simulink model "BlokSchema3 - Older"  (R2022a)
settings: Solver=VariableStepAuto  StartTime=0.0  StopTime=5000  RelTol=1e-5
values from neighbouring files (symbols this model uses):
  citatel = (K/(T1*T2))    (= 0.00186096256684)    [Zadanie3.m]    (also in Zadanie3_v2.m)
  Delay = 300    [Zadanie3.m]    (also in Zadanie3_v2.m)
  menovatel = [1,(T1+T2)/(T1*T2), 1/(T1*T2)]    [Zadanie3.m]    (also in Zadanie3_v2.m)
  p01 = citatel1(2)*q00    [Zadanie3.m]    (also in Zadanie3_v2.m)
  p02 = citatel1(3)*q00    [Zadanie3.m]    (also in Zadanie3_v2.m)
  p03 = citatel1(4)*q00    [Zadanie3_v2.m]
  p11 = q10*citatel1(2)    [Zadanie3.m]    (also in Zadanie3_v2.m)
  p12 = q10*(citatel1(3)-citatel1(2))+(citatel1(2)/bSum)    [Zadanie3.m]    (also in Zadanie3_v2.m)
  p13 = q10*(citatel1(4)-citatel1(3))+(citatel1(3)/bSum)    [Zadanie3.m]    (also in Zadanie3_v2.m)
  q00 = 1/sum(citatel1(2:end))    [Zadanie3.m]    (also in Zadanie3_v2.m)
  q01 = menovatel1(2)*q00    [Zadanie3.m]    (also in Zadanie3_v2.m)
  q02 = menovatel1(3)*q00    [Zadanie3.m]    (also in Zadanie3_v2.m)
  q03 = menovatel1(4)*q00    [Zadanie3_v2.m]
  q10 = 0.089115984    [Zadanie3.m]    (also in Zadanie3_v2.m)
  q11 = q10*(menovatel1(2)-1)+1/bSum    [Zadanie3.m]    (also in Zadanie3_v2.m)
  q12 = q10*(menovatel1(3)-menovatel1(2))+(menovatel1(2)/bSum)    [Zadanie3.m]    (also in Zadanie3_v2.m)
  q13 = q10*(menovatel1(4)-menovatel1(3))+(menovatel1(3)/bSum)    [Zadanie3.m]    (also in Zadanie3_v2.m)
  T = 300    [Zadanie3.m]    (also in Zadanie3_v2.m)
settings Model: PacingRate=100  Creator=domin  LastModifiedBy=domin
settings ModelReferenceCC: EnableRefExpFcnMdlSchedulingChecks=off
settings RTWCC: Description=Generic Real-Time Target

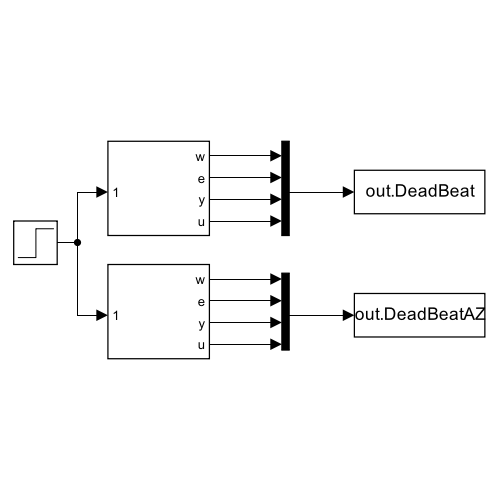
[thumbnail: Simulink's stored preview of the top-level diagram]
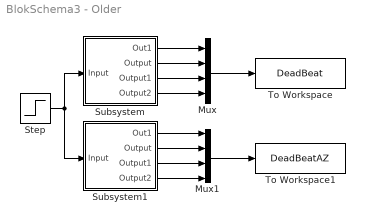
== system BlokSchema3 - Older ==
  Mux : Mux
  Mux1 : Mux
  Step : Step  Time=0  Before=1  SampleTime=0
  Subsystem : Subsystem
  Subsystem1 : Subsystem
  To Workspace : ToWorkspace  VariableName=DeadBeat  SaveFormat=Timeseries  SampleTime=-1
  To Workspace1 : ToWorkspace  VariableName=DeadBeatAZ  SaveFormat=Timeseries  SampleTime=-1
  wires:
  Step/1 -> Subsystem/1(Input), Subsystem1/1(Input)
  Subsystem/1(Out1) -> Mux/1
  Subsystem/2(Output) -> Mux/2
  Subsystem/3(Output1) -> Mux/3
  Subsystem/4(Output2) -> Mux/4
  Mux/1 -> To Workspace/1
  Mux1/1 -> To Workspace1/1
  Subsystem1/1(Out1) -> Mux1/1
  Subsystem1/2(Output) -> Mux1/2
  Subsystem1/3(Output1) -> Mux1/3
  Subsystem1/4(Output2) -> Mux1/4

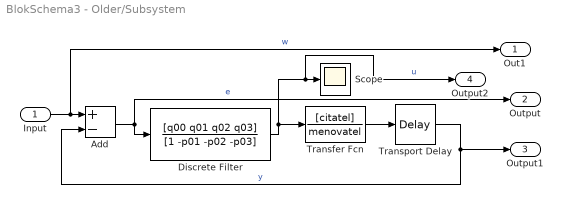
== system BlokSchema3 - Older/Subsystem ==
  Input : Inport
  Add : Sum  Inputs=+-
  Discrete Filter : DiscreteFilter  Numerator=[q00 q01 q02 q03]  Denominator=[1 -p01 -p02 -p03]  SampleTime=T
  Scope : Scope
  Transfer Fcn : TransferFcn  Numerator=[citatel]  Denominator=menovatel
  Transport Delay : TransportDelay  DelayTime=Delay
  Out1 : Outport
  Output : Outport  Port=2
  Output1 : Outport  Port=3
  Output2 : Outport  Port=4
  wires:
  Add/1 -> Output/1, Discrete Filter/1  "e"
  Input/1 -> Out1/1, Add/1  "w"
  Transfer Fcn/1 -> Transport Delay/1
  Discrete Filter/1 -> Transfer Fcn/1, Output2/1, Scope/1  "u"
  Transport Delay/1 -> Output1/1, Add/2  "y"

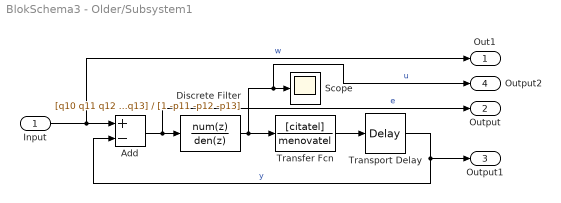
== system BlokSchema3 - Older/Subsystem1 ==
  Input : Inport
  Add : Sum  Inputs=+-
  Discrete Filter : DiscreteFilter  Numerator=[q10 q11 q12 q13]  Denominator=[1 -p11 -p12 -p13]  SampleTime=T
  Scope : Scope
  Transfer Fcn : TransferFcn  Numerator=[citatel]  Denominator=menovatel
  Transport Delay : TransportDelay  DelayTime=Delay
  Out1 : Outport
  Output : Outport  Port=2
  Output1 : Outport  Port=3
  Output2 : Outport  Port=4
  wires:
  Add/1 -> Discrete Filter/1, Output/1  "e"
  Input/1 -> Out1/1, Add/1  "w"
  Transfer Fcn/1 -> Transport Delay/1
  Discrete Filter/1 -> Transfer Fcn/1, Output2/1, Scope/1  "u"
  Transport Delay/1 -> Output1/1, Add/2  "y"
